simulink model "FurutaPendulum_EnesUslu"  (R2018b)
settings: Solver=FixedStepAuto  StartTime=0.0  StopTime=10.0  FixedStep=Ts  RelTol=1e-3
values from neighbouring files (symbols this model uses):
  dTheta0_init = 0    [FurutaPendulum_Constants.m]
  dTheta1_init = 0    [FurutaPendulum_Constants.m]
  Theta0_init = -pi/2    (= -1.57079632679)    [FurutaPendulum_Constants.m]
  Theta1_init = 2.5*pi/3    (= 2.61799387799)    [FurutaPendulum_Constants.m]
undefined symbols (not defined in the file or in its folder): K1
libraries: simulink_extras x1
settings Model: Creator=PC  LastModifiedBy=PC
settings DebuggingCC: ParameterOverflowMsg=warning  UnderSpecifiedDimensionMsg=warning

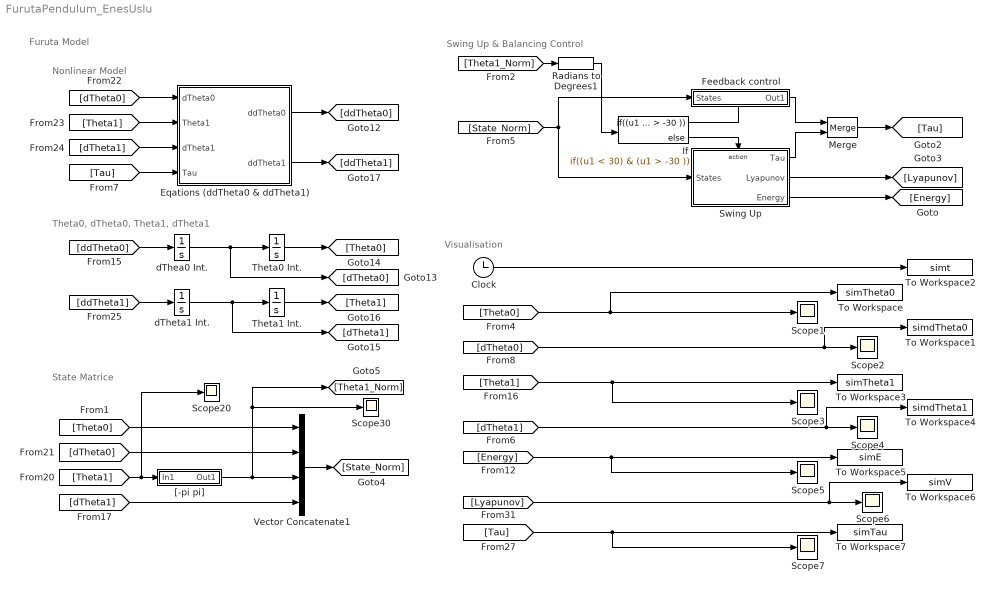
== system FurutaPendulum_EnesUslu ==
  note: Visualisation
  note: Swing Up & Balancing Control
  note: Nonlinear Model
  note: Theta0, dTheta0, Theta1, dTheta1
  note: State Matrice
  note: Furuta Model
  " dThea0 Int." : Integrator  InitialCondition=dTheta0_init
  Clock : Clock
  Eqations (ddTheta0 & ddTheta1) : MATLAB Function  TreatAsAtomicUnit=on
  Feedback control : Subsystem  TreatAsAtomicUnit=on
  If : If  IfExpression=(u1 < 30) & (u1 > -30 )
  Merge : Merge
  Radians to Degrees1 : simulink_extras/Transformations/Radians to Degrees
  Scope{1..7,20,30} (9 alike) : Scope
  Swing Up : Subsystem  TreatAsAtomicUnit=on
  Theta0 Int. : Integrator  InitialCondition=Theta0_init
  Theta1 Int. : Integrator  InitialCondition=Theta1_init
  To Workspace : ToWorkspace  VariableName=simTheta0  SampleTime=-1
      settings: Save2DSignal=2-D array (concatenate along first dimension)
  To Workspace1 : ToWorkspace  VariableName=simdTheta0  SampleTime=-1
      settings: Save2DSignal=2-D array (concatenate along first dimension)
  To Workspace2 : ToWorkspace  VariableName=simt  SampleTime=-1
      settings: Save2DSignal=2-D array (concatenate along first dimension)
  To Workspace3 : ToWorkspace  VariableName=simTheta1  SampleTime=-1
      settings: Save2DSignal=2-D array (concatenate along first dimension)
  To Workspace4 : ToWorkspace  VariableName=simdTheta1  SampleTime=-1
      settings: Save2DSignal=2-D array (concatenate along first dimension)
  To Workspace5 : ToWorkspace  VariableName=simE  SampleTime=-1
      settings: Save2DSignal=2-D array (concatenate along first dimension)
  To Workspace6 : ToWorkspace  VariableName=simV  SampleTime=-1
      settings: Save2DSignal=2-D array (concatenate along first dimension)
  To Workspace7 : ToWorkspace  VariableName=simTau  SampleTime=-1
      settings: Save2DSignal=2-D array (concatenate along first dimension)
  Vector Concatenate1 : Concatenate  NumInputs=4
  "[-pi pi]" : Subsystem
  dTheta1 Int. : Integrator  InitialCondition=dTheta1_init
  wires:
  [Theta1] -> Eqations (ddTheta0 & ddTheta1)/2(Theta1)
  Eqations (ddTheta0 & ddTheta1)/1(ddTheta0) -> [ddTheta0]
  Theta1 Int./1 -> [Theta1]
  Feedback control/1(Out1) -> Merge/1
  Theta0 Int./1 -> [Theta0]
  Radians to Degrees1/1 -> If/1
  [Theta1_Norm] -> Radians to Degrees1/1
  [dTheta0] -> Eqations (ddTheta0 & ddTheta1)/1(dTheta0)
  If/1 -> Feedback control/Action
  [Theta0] -> Scope1/1, To Workspace/1
  Clock/1 -> To Workspace2/1
  dTheta1 Int./1 -> [dTheta1], Theta1 Int./1
  "[-pi pi]"/1(Out1) -> [Theta1_Norm], Scope30/1, Vector Concatenate1/3
  [dTheta0] -> Scope2/1, To Workspace1/1
  Swing Up/2(Lyapunov) -> [Lyapunov]
  Merge/1 -> [Tau]
  [dTheta1] -> Eqations (ddTheta0 & ddTheta1)/3(dTheta1)
  [Theta1] -> Scope20/1, "[-pi pi]"/1(In1)
  Swing Up/3(Energy) -> [Energy]
  [ddTheta1] -> dTheta1 Int./1
  [Tau] -> Eqations (ddTheta0 & ddTheta1)/4(Tau)
  [ddTheta0] -> " dThea0 Int."/1
  [dTheta1] -> Scope4/1, To Workspace4/1
  [dTheta1] -> Vector Concatenate1/4
  [State_Norm] -> Feedback control/1(States), Swing Up/1(States)
  Swing Up/1(Tau) -> Merge/2
  [Tau] -> To Workspace7/1, Scope7/1
  [Theta1] -> To Workspace3/1, Scope3/1
  [Energy] -> To Workspace5/1, Scope5/1
  Eqations (ddTheta0 & ddTheta1)/2(ddTheta1) -> [ddTheta1]
  [Lyapunov] -> Scope6/1, To Workspace6/1
  If/2 -> Swing Up/Action
  [Theta0] -> Vector Concatenate1/1
  [dTheta0] -> Vector Concatenate1/2
  " dThea0 Int."/1 -> [dTheta0], Theta0 Int./1
  Vector Concatenate1/1 -> [State_Norm]

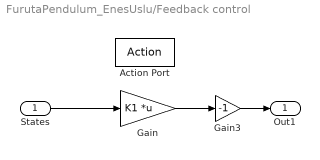
== system FurutaPendulum_EnesUslu/Feedback control ==
  States : Inport
  Action Port : ActionPort  ActionType=then
  Gain : Gain  Gain=K1  Multiplication=Matrix(K*u)  ParamDataTypeStr=double  OutDataTypeStr=double
  Gain3 : Gain  Gain=-1
  Out1 : Outport
  wires:
  States/1 -> Gain/1
  Gain/1 -> Gain3/1
  Gain3/1 -> Out1/1

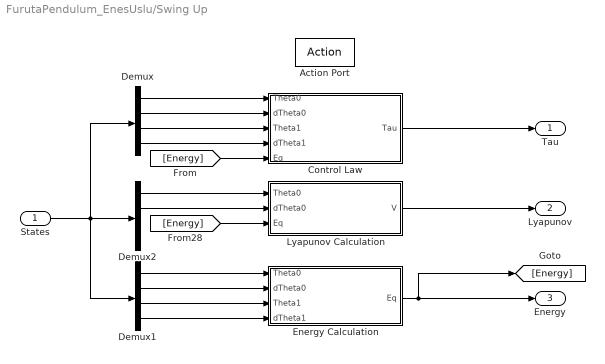
== system FurutaPendulum_EnesUslu/Swing Up ==
  States : Inport
  Action Port : ActionPort  ActionType=else
  Control Law : MATLAB Function  TreatAsAtomicUnit=on
  Demux : Demux
  Demux1 : Demux
  Demux2 : Demux
  Energy Calculation : MATLAB Function  TreatAsAtomicUnit=on
  Lyapunov Calculation : MATLAB Function  TreatAsAtomicUnit=on
  Tau : Outport  InitialOutput=0
  Lyapunov : Outport  Port=2  InitialOutput=0
  Energy : Outport  Port=3  InitialOutput=0
  wires:
  Control Law/1(Tau) -> Tau/1
  Demux/3 -> Control Law/3(Theta1)
  Demux/4 -> Control Law/4(dTheta1)
  Lyapunov Calculation/1(V) -> Lyapunov/1
  Demux/1 -> Control Law/1(Theta0)
  Demux/2 -> Control Law/2(dTheta0)
  States/1 -> Demux/1, Demux1/1, Demux2/1
  Energy Calculation/1(Eq) -> Energy/1, [Energy]
  Demux1/1 -> Energy Calculation/1(Theta0)
  Demux1/2 -> Energy Calculation/2(dTheta0)
  Demux1/3 -> Energy Calculation/3(Theta1)
  Demux1/4 -> Energy Calculation/4(dTheta1)
  [Energy] -> Control Law/5(Eq)
  Demux2/1 -> Lyapunov Calculation/1(Theta0)
  Demux2/2 -> Lyapunov Calculation/2(dTheta0)
  [Energy] -> Lyapunov Calculation/3(Eq)

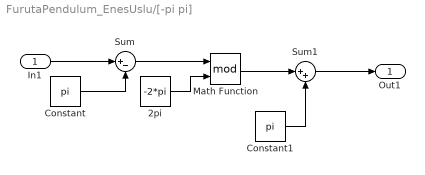
== system FurutaPendulum_EnesUslu/[-pi pi] ==
  In1 : Inport
  2pi : Constant  Value=-2*pi
  Constant : Constant  Value=pi
  Constant1 : Constant  Value=pi
  Math Function : Math  Operator=mod  SaturateOnIntegerOverflow=on
  Sum : Sum  Inputs=|+-
  Sum1 : Sum  Inputs=|++
  Out1 : Outport
  wires:
  2pi/1 -> Math Function/2
  In1/1 -> Sum/1
  Sum/1 -> Math Function/1
  Constant/1 -> Sum/2
  Constant1/1 -> Sum1/2
  Sum1/1 -> Out1/1
  Math Function/1 -> Sum1/1

== matlab function FurutaPendulum_EnesUslu/Eqations (ddTheta0 & ddTheta1) ==
  data: dTheta0 input; Theta1 input; dTheta1 input; ddTheta0 output; Tau input; ddTheta1 output
function [ddTheta0,ddTheta1] = fcn(dTheta0, Theta1, dTheta1, Tau)
%% Constants 0 - Arm 1 - Pendulum 
I0=1.75*10^-2;      %Inertia of the arm (kg*m^2)
L0=0.215;           %Total length of the arm  (m)
m1=5.38*10^-2;      %Mass of the pendulum (kg)
L1=0.113;           %Distance to the center of gravity of the pendulum (m)
J1=1.98*10^-4;      %Inertia of the pendulum around its center of gravity (kg*m^2)
%Theta0=0.001;      %Rotational angle of the arm
%Theta1=0.001;      %Rotational angle of the pendulum
%tau=0.071;         %Input torque applied on the arm
g = 9.81;           %Gravity (m/s^2)
%% D(q)
%ddTheta0 = 0;
Dq=[I0+m1*(L0^2+L1^2*(sin(Theta1))^2) m1*L1*L0*cos(Theta1); m1*L1*L0*cos(Theta1) J1+m1*L1^2];
%% ddTheta0 & ddTheta1
ddTheta0 = (1/det(Dq))*((J1+m1*L1^2)*Tau - ...
    (J1+m1*L1^2)*m1*L1^2*sin(2*Theta1)*dTheta0*dTheta1-...
    (1/2)*m1^2*L1^3*L0*cos(Theta1)*sin(2*Theta1)*dTheta0^2 + ...
    (J1+m1*L1^2)*m1*L1*L0*sin(Theta1)*dTheta1^2 - ...
    m1^2*L1^2*L0*g*cos(Theta1)*sin(Theta1));
ddTheta1 = (1/det(Dq))*(...
    -1*(m1*L1*L0*cos(Theta1))*Tau - ...
    m1^2*L1^2*L0^2*sin(Theta1)*cos(Theta1)*dTheta1^2 + ...
    m1*L1^2*sin(2*Theta1)*dTheta0*(...
    m1*L1*L0*cos(Theta1)*dTheta1 + ...
    (1/2)*(I0+m1*L0^2 + L1^2*(sin(Theta1))^2)*dTheta0) + ...
    (I0+m1*L0^2 + L1^2*(sin(Theta1))^2)*m1*L1*g*sin(Theta1)...
    );

% u=[Theta1;dTheta1; dTheta0; Tau; -4.7940e-04*dTheta1]
% m0 = 0.380; 
% M = 0.044;
% alpha = J1 + (M+m0/3+m1)*L0^2;
% beta = (M + m1/3)*L1^2;
% gamma = (M + m1/2)*L1*L0;
% sigma = (M + m1/2)*g*L1;
% ddTheta1=((beta*(alpha+beta*sin(u(1))*sin(u(1)))*cos(u(1))*sin(u(1))*u(3)*u(3))+(2*beta*gamma*(1-sin(u(1))*sin(u(1)))*sin(u(1))*u(3)*u(2))-(gamma*gamma*cos(u(1))*sin(u(1))*u(2)*u(2))+(sigma*(alpha+beta*sin(u(1))*sin(u(1)))*sin(u(1)))-(gamma*cos(u(1))*u(4))+((alpha+beta*sin(u(1))*sin(u(1)))*u(5)))/...
%     ((alpha*beta)-(gamma*gamma)+((beta*beta+gamma*gamma)*sin(u(1))*sin(u(1))));

== matlab function FurutaPendulum_EnesUslu/Swing Up/Control Law ==
  data: Theta0 input; dTheta0 input; Tau output; Theta1 input; dTheta1 input; Eq input
function Tau  = fcn(Theta0, dTheta0, Theta1, dTheta1, Eq)
%% Constants 0 - Arm 1 - Pendulum 
I0=1.75*10^-2;      %Inertia of the arm (kg*m^2)
L0=0.215;           %Total length of the arm  (m)
m1=5.38*10^-2;      %Mass of the pendulum (kg)
L1=0.113;           %Distance to the center of gravity of the pendulum (m)
J1=1.98*10^-4;      %Inertia of the pendulum around its center of gravity (kg*m^2)
%Theta0=0.001;      %Rotational angle of the arm
%Theta1=0.001;      %Rotational angle of the pendulum
%tau=0.071;         %Input torque applied on the arm
g = 9.81;           %Gravity (m/s^2)

% kE = 480;
kE = 480
kth = 1;
kw = 1;
kd = 1;
k = 6; %1 1: for oscillation, 6: for state feedback condition to be achieved
%% D(q)
%ddTheta0 = 0;
% Dq = 0
Dq=[I0+m1*(L0^2+L1^2*(sin(Theta1))^2) m1*L1*L0*cos(Theta1); m1*L1*L0*cos(Theta1) J1+m1*L1^2];
% Fq = 0
Fq = (...
    -(J1+m1*L1^2)*m1*L1^2*sin(2*Theta1)*dTheta0*dTheta1-(1/2)*m1^2*L1^3*L0*cos(Theta1)*sin(2*Theta1)*dTheta0^2 + ...
    (J1+m1*L1^2)*m1*L1*L0*sin(Theta1)*dTheta1^2 - m1^2*L1^2*L0*g*cos(Theta1)*sin(Theta1)...
    );
% Tau = 0;
Tau = k*(-kw*Fq - det(Dq)*(kd*dTheta0+kth*Theta0))/(det(Dq)*kE*Eq + kw*(J1+m1*L1^2));

== matlab function FurutaPendulum_EnesUslu/Swing Up/Energy Calculation ==
  data: Theta0 input; Eq output; dTheta0 input; Theta1 input; dTheta1 input
function Eq  = fcn(Theta0, dTheta0, Theta1, dTheta1)
%% Constants 0 - Arm 1 - Pendulum 
I0=1.75*10^-2;      %Inertia of the arm (kg*m^2)
L0=0.215;           %Total length of the arm  (m)
m1=5.38*10^-2;      %Mass of the pendulum (kg)
L1=0.113;           %Distance to the center of gravity of the pendulum (m)
J1=1.98*10^-4;      %Inertia of the pendulum around its center of gravity (kg*m^2)
%Theta0=0.001;      %Rotational angle of the arm
%Theta1=0.001;      %Rotational angle of the pendulum
%tau=0.071;         %Input torque applied on the arm
g = 9.81;           %Gravity (m/s^2)
 
% state(1,1)= Theta0;
% state(1,2)= dTheta0;
% state(1,3)= Theta1;
% state(1,4)= dTheta1;

%% E(q) = K(q,dq) + P(q)
Dq=[I0+m1*(L0^2+L1^2*(sin(Theta1))^2) m1*L1*L0*cos(Theta1); m1*L1*L0*cos(Theta1) J1+m1*L1^2];
dq =[dTheta0; dTheta1];
Eq = (1/2)*transpose(dq)*Dq*dq + m1*g*L1*(cos(Theta1)-1);

== matlab function FurutaPendulum_EnesUslu/Swing Up/Lyapunov Calculation ==
  data: Theta0 input; dTheta0 input; V output; Eq input
function V  = fcn(Theta0, dTheta0, Eq)
kE = 480;
kth = 1;
kw = 1;
V = (kE/2)*Eq^2 + (kw/2)*(dTheta0)^2 + (kth/2)*Theta0^2;
